simulink model "adaptive_control_new"  (R2023b)
settings: Solver=VariableStepAuto  StartTime=0.0  StopTime=tf  RelTol=1e-8
values from neighbouring files (symbols this model uses):
  A = Ixx-Kpdot    (= 4100300)    [ShipFinStabilizers.m]
  alpha = 100000    [ShipFinStabilizers.m]
  Am = [0 1; -16/ts^2, -8/ts]    [ShipFinStabilizers.m]
  B = Kp + Kup - 2*Kalpha*rf/U    (= -510163.123)    [ShipFinStabilizers.m]
  beta = alpha/100    (= 1000)    [ShipFinStabilizers.m]
  Bm = [0; 16/ts^2]    [ShipFinStabilizers.m]
  C = Knl    (= -416000)    [ShipFinStabilizers.m]
  controller_on = 0    [off.m]    (also in on.m = 1; plotRoutine.m)
  D = KphiUU*U^2    (= -265500)    [ShipFinStabilizers.m]
  F = -2*Kalpha    (= -36069.75)    [ShipFinStabilizers.m]
  Fw = 0    [ShipFinStabilizers.m]    (also in plotRoutine.m = 0.1)
  omega_w = 1.3    [ShipFinStabilizers.m]    (also in plotRoutine.m)
  sat = 20    [ShipFinStabilizers.m]
  x0 = [0;0]    [ShipFinStabilizers.m]    (also in plotRoutine.m = [deg2rad(10);0])
libraries: eeGeneralControl x1, simulink x1
settings Model: Creator=valen  LastModifiedBy=valen

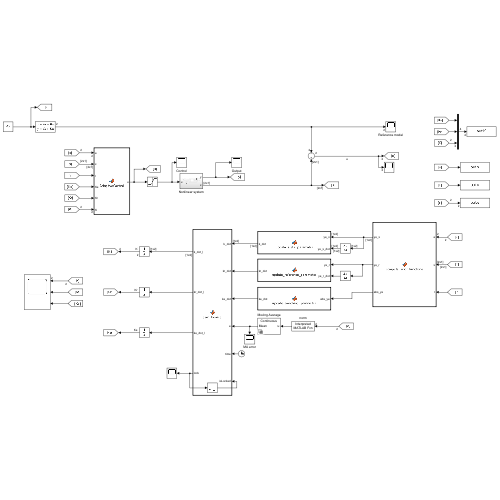
[thumbnail: Simulink's stored preview of the top-level diagram]
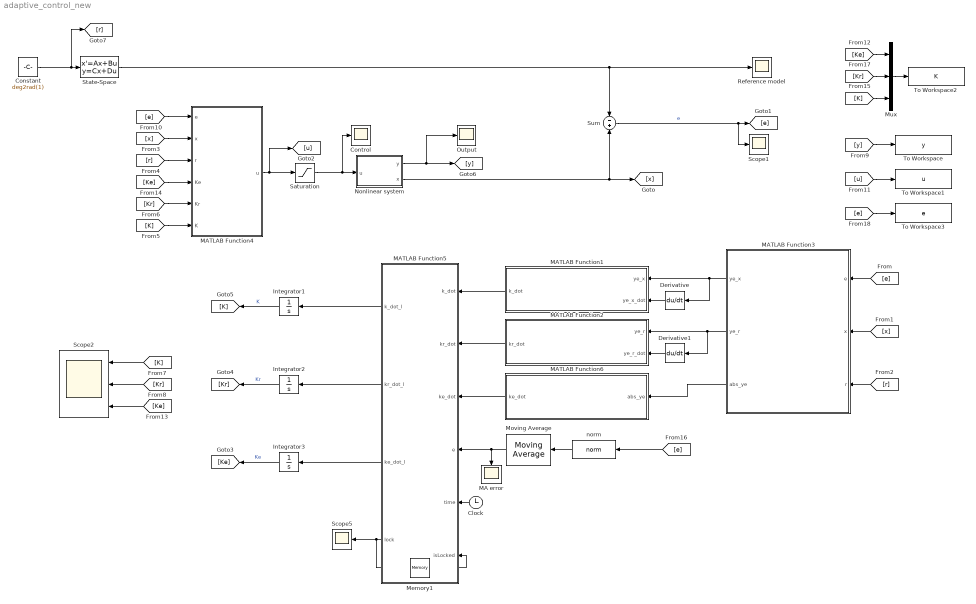
== system adaptive_control_new ==
  Clock : Clock
  Constant : Constant  Value=deg2rad(1)
  Control : Scope
  Derivative : Derivative
  Derivative1 : Derivative
  Integrator1 : Integrator  InitialCondition=[0,0]
  Integrator2 : Integrator
  Integrator3 : Integrator
  MA error : Scope
  MATLAB Function1 : MATLAB Function  TreatAsAtomicUnit=on
  MATLAB Function2 : MATLAB Function  TreatAsAtomicUnit=on
  MATLAB Function3 : MATLAB Function  TreatAsAtomicUnit=on
  MATLAB Function4 : MATLAB Function  TreatAsAtomicUnit=on
  MATLAB Function5 : MATLAB Function  TreatAsAtomicUnit=on
  MATLAB Function6 : MATLAB Function  TreatAsAtomicUnit=on
  Memory1 : Memory
  Moving Average : eeGeneralControl/Moving Average  VariantControl=Variant1  LabelModeActiveChoice=Continuous  f=1/10  x0=0  BufferSize=8192  Ts=0
      settings: LibrarySourceBlock=ee_sl_lib/General Control/Moving Average
  Mux : Mux  Inputs=3
  Nonlinear system : Subsystem
  Output : Scope
  Reference model : Scope
  Saturation : Saturate  UpperLimit=sat  LowerLimit=-sat
  Scope1 : Scope
  Scope2 : Scope  NumInputPorts=3
  Scope5 : Scope
  State-Space : StateSpace  A=Am  B=Bm  C=eye(2)  D=[0;0]  InitialCondition=x0
  Sum : Sum  Inputs=-+
  To Workspace : ToWorkspace  VariableName=y  SaveFormat=Timeseries  SampleTime=-1
  To Workspace1 : ToWorkspace  VariableName=u  SaveFormat=Timeseries  SampleTime=-1
  To Workspace2 : ToWorkspace  VariableName=K  SaveFormat=Timeseries  SampleTime=-1
  To Workspace3 : ToWorkspace  VariableName=e  SaveFormat=Timeseries  SampleTime=-1
  norm : MATLABFcn  MATLABFcn=norm
  wires:
  Nonlinear system/2(x) -> [x], Sum/2
  Sum/1 -> [e], Scope1/1  "e"
  [r] -> MATLAB Function3/3(r)
  [e] -> MATLAB Function3/1(e)
  [x] -> MATLAB Function3/2(x)
  MATLAB Function3/3(abs_ye) -> MATLAB Function6/1(abs_ye)
  MATLAB Function3/2(ye_r) -> Derivative1/1, MATLAB Function2/1(ye_r)
  Derivative/1 -> MATLAB Function1/2(ye_x_dot)
  Derivative1/1 -> MATLAB Function2/2(ye_r_dot)
  MATLAB Function3/1(ye_x) -> Derivative/1, MATLAB Function1/1(ye_x)
  Memory1/1 -> MATLAB Function5/6(isLocked)
  MATLAB Function5/4(lock) -> Memory1/1, Scope5/1
  Integrator1/1 -> [K]  "K"
  Integrator2/1 -> [Kr]  "Kr"
  Integrator3/1 -> [Ke]  "Ke"
  MATLAB Function4/1(u) -> [u], Saturation/1
  [x] -> MATLAB Function4/2(x)
  [r] -> MATLAB Function4/3(r)
  [K] -> MATLAB Function4/6(K)
  [Kr] -> MATLAB Function4/5(Kr)
  [K] -> Scope2/1
  [Kr] -> Scope2/2
  Nonlinear system/1(y) -> [y], Output/1
  [Ke] -> MATLAB Function4/4(Ke)
  [e] -> MATLAB Function4/1(e)
  [Ke] -> Scope2/3
  Saturation/1 -> Nonlinear system/1(u), Control/1
  MATLAB Function1/1(k_dot) -> MATLAB Function5/1(k_dot)
  MATLAB Function2/1(kr_dot) -> MATLAB Function5/2(kr_dot)
  MATLAB Function5/1(k_dot_l) -> Integrator1/1
  MATLAB Function5/2(kr_dot_l) -> Integrator2/1
  MATLAB Function5/3(ke_dot_l) -> Integrator3/1
  norm/1 -> Moving Average/1
  [e] -> norm/1
  Constant/1 -> [r], State-Space/1
  Clock/1 -> MATLAB Function5/5(time)
  Moving Average/1 -> MA error/1, MATLAB Function5/4(e)
  [y] -> To Workspace/1
  [u] -> To Workspace1/1
  [Kr] -> Mux/2
  [Ke] -> Mux/1
  [K] -> Mux/3
  Mux/1 -> To Workspace2/1
  [e] -> To Workspace3/1
  State-Space/1 -> Reference model/1, Sum/1
  MATLAB Function6/1(ke_dot) -> MATLAB Function5/3(ke_dot)

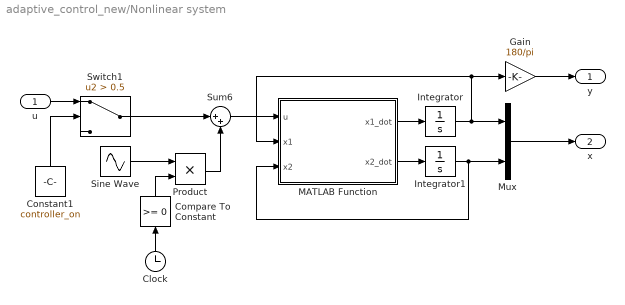
== system adaptive_control_new/Nonlinear system ==
  u : Inport
  Clock : Clock
  Compare To Constant : simulink/Logic and Bit Operations/Compare To Constant  relop=>=  const=0  OutDataTypeStr=boolean
  Constant1 : Constant  Value=controller_on
  Gain : Gain  Gain=180/pi
  Integrator : Integrator  InitialCondition=x0(1)
  Integrator1 : Integrator  InitialCondition=x0(2)
  MATLAB Function : MATLAB Function  TreatAsAtomicUnit=on
  Mux : Mux  Inputs=2
  Product : Product
  Sine Wave : Sin  Amplitude=Fw/F*A  Frequency=omega_w  SampleTime=0
  Sum6 : Sum  Inputs=|++
  Switch1 : Switch  Criteria=u2 > Threshold  Threshold=0.5  SaturateOnIntegerOverflow=off  InputSameDT=off
  y : Outport
  x : Outport  Port=2
  wires:
  Integrator1/1 -> Mux/2, MATLAB Function/3(x2)
  Integrator/1 -> Mux/1, Gain/1, MATLAB Function/2(x1)
  MATLAB Function/2(x2_dot) -> Integrator1/1
  MATLAB Function/1(x1_dot) -> Integrator/1
  Constant1/1 -> Switch1/2
  Sine Wave/1 -> Product/1
  Switch1/1 -> Sum6/1
  Product/1 -> Sum6/2
  Compare To Constant/1 -> Product/2
  Clock/1 -> Compare To Constant/1
  Sum6/1 -> MATLAB Function/1(u)
  u/1 -> Switch1/1
  Gain/1 -> y/1
  Mux/1 -> x/1

== matlab function adaptive_control_new/MATLAB Function1 ==
  data: ye_x input; k_dot output size=[1,2]; ye_x_dot input; alpha parameter; beta parameter
function k_dot = update_state_parameter(ye_x, ye_x_dot, alpha, beta)


k_dot = alpha*ye_x + beta *ye_x_dot;

== matlab function adaptive_control_new/Nonlinear system/MATLAB Function ==
  data: u input; x1_dot output; x1 input; x2 input; x2_dot output; A parameter; B parameter; C parameter; D parameter; E parameter; F parameter
function [x1_dot,x2_dot] = ship(u,x1,x2, A, B, C, D, E, F)

    x1_dot = x2;
    x2_dot = 1/A*( B*x2 + C*x2*abs(x2) + D*x1 + E*sin(x1) + F*u);

== matlab function adaptive_control_new/MATLAB Function2 ==
  data: ye_r input; kr_dot output; ye_r_dot input; alpha parameter; beta parameter
function kr_dot = update_reference_parameter(ye_r, ye_r_dot, alpha, beta)


kr_dot = alpha*ye_r + beta *ye_r_dot;

== matlab function adaptive_control_new/MATLAB Function3 ==
  data: e input; x input; r input; ye_x output; ye_r output; Ce parameter; abs_ye output
function [ye_x, ye_r,abs_ye] = compute_error_functions(e, x, r, Ce)
ye = Ce*e;
ye_x = ye*x';
ye_r = ye*r';
abs_ye = abs(ye);

== matlab function adaptive_control_new/MATLAB Function4 ==
  data: e input; x input size=[2;1]; r input; Ke input; Kr input; K input; u output; Ce parameter
function u = AdaptiveControl(e, x, r,Ke, Kr, K, Ce)

u = -(Kr*r + K(1)*x(1) + K(2)*x(2)) + Ke*tanh([1, 1]*e);

end

function s = reg_sign(e)

    if norm(e)<1
        s = e;
    else
        s=sign(e);
    end
end

== matlab function adaptive_control_new/MATLAB Function5 ==
  data: k_dot input; k_dot_l output; kr_dot input; ke_dot input; e input; time input; kr_dot_l output; ke_dot_l output; lock output; isLocked input; gain_locking_start parameter
function [k_dot_l, kr_dot_l,ke_dot_l, lock] = gain_locking(k_dot,kr_dot, ke_dot,e, time, isLocked,gain_locking_start)


if (norm(e) < 2e-3 || isLocked) && time>gain_locking_start
    k_dot_l = zeros(1,2);
    kr_dot_l = 0;
    ke_dot_l = 0;
    lock = 1;
else
    k_dot_l = k_dot;
    kr_dot_l = kr_dot;
    ke_dot_l = ke_dot;
    lock = 0;
end

== matlab function adaptive_control_new/MATLAB Function6 ==
  data: abs_ye input; ke_dot output; gamma parameter
function ke_dot = update_switching_parameter(abs_ye,gamma)


ke_dot = gamma*abs_ye;
